simulink model "gauges"  (Simulink 7.5)
settings: Solver=ode45  StartTime=0.0  StopTime=10.0  RelTol=1e-3
undefined symbols (not defined in the file or in its folder): ECU565, motohawk_get_faults
libraries: MotoHawk_VDOGauge_lib x6, MotoHawk_lib x4, simulink x1
settings Model: Creator=Ethan  LastModifiedBy=Ethan

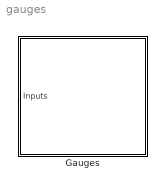
== system gauges ==
  Gauges : Subsystem

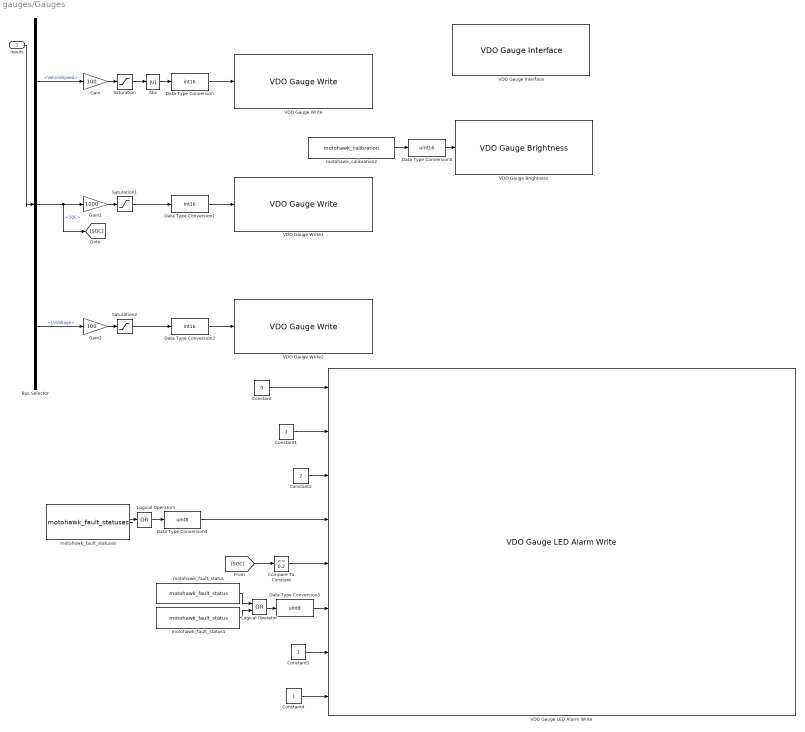
== system gauges/Gauges ==
  Inputs : Inport  OutDataType=sfix(16)  OutScaling=2^0
  Abs : Abs  OutDataType=fixdt(1, 16)  OutScaling=2^0
  Bus Selector : BusSelector  OutputSignals=VehicleSpeed,SOC,LVVoltage
  Compare To Constant : simulink/Logic and Bit Operations/Compare To Constant  SystemSampleTime=-1  relop=<=  const=0.2  LogicOutDataTypeMode=uint8
  Constant : Constant  Value=0  OutDataTypeMode=uint8  OutDataType=fixdt(1, 16)  OutScaling=2^0  OutDataTypeStr=uint8
  Constant1 : Constant  OutDataTypeMode=uint8  OutDataType=fixdt(1, 16)  OutScaling=2^0  OutDataTypeStr=uint8
  Constant2 : Constant  Value=2  OutDataTypeMode=uint8  OutDataType=fixdt(1, 16)  OutScaling=2^0  OutDataTypeStr=uint8
  Constant3 : Constant  OutDataTypeMode=uint8  OutDataType=fixdt(1, 16)  OutScaling=2^0  OutDataTypeStr=uint8
  Constant4 : Constant  OutDataTypeMode=uint8  OutDataType=fixdt(1, 16)  OutScaling=2^0  OutDataTypeStr=uint8
  Data Type Conversion : DataTypeConversion  OutDataTypeMode=int16  OutDataType=fixdt(1, 16)  OutScaling=2^0  OutDataTypeStr=int16
  Data Type Conversion1 : DataTypeConversion  OutDataTypeMode=int16  OutDataType=fixdt(1, 16)  OutScaling=2^0  OutDataTypeStr=int16
  Data Type Conversion2 : DataTypeConversion  OutDataTypeMode=int16  OutDataType=fixdt(1, 16)  OutScaling=2^0  OutDataTypeStr=int16
  Data Type Conversion3 : DataTypeConversion  OutDataTypeMode=uint8  OutDataType=fixdt(1, 16)  OutScaling=2^0  OutDataTypeStr=uint8
  Data Type Conversion4 : DataTypeConversion  OutDataTypeMode=uint8  OutDataType=fixdt(1, 16)  OutScaling=2^0  OutDataTypeStr=uint8
  Data Type Conversion5 : DataTypeConversion  OutDataTypeMode=uint16  OutDataType=fixdt(1, 16)  OutScaling=2^0  OutDataTypeStr=uint16
  Gain : Gain  Gain=100  ParameterDataType=fixdt(1, 16)  ParameterScaling=2^0  OutDataType=fixdt(1, 16)  OutScaling=2^0
  Gain1 : Gain  Gain=1000  ParameterDataType=fixdt(1, 16)  ParameterScaling=2^0  OutDataType=fixdt(1, 16)  OutScaling=2^0
  Gain2 : Gain  Gain=100  ParameterDataType=fixdt(1, 16)  ParameterScaling=2^0  OutDataType=fixdt(1, 16)  OutScaling=2^0
  Logical Operator : Logic  Operator=OR  AllPortsSameDT=off  OutDataTypeMode=boolean  LogicDataType=fixdt(0, 8)  OutDataTypeStr=boolean
  Logical Operator1 : Logic  Operator=OR  Inputs=1  AllPortsSameDT=off  OutDataTypeMode=boolean  LogicDataType=fixdt(0, 8)  OutDataTypeStr=boolean
  Saturation : Saturate  UpperLimit=100  LowerLimit=-100  OutDataType=fixdt(1, 16)  OutScaling=2^0
  Saturation1 : Saturate  UpperLimit=1000  LowerLimit=0  OutDataType=fixdt(1, 16)  OutScaling=2^0
  Saturation2 : Saturate  UpperLimit=20  LowerLimit=0  OutDataType=fixdt(1, 16)  OutScaling=2^0
  VDO Gauge Brightness : MotoHawk_VDOGauge_lib/VDO Gauge Brightness  nam='GaugeChain'  per=2000
  VDO Gauge Interface : MotoHawk_VDOGauge_lib/VDO Gauge Interface  nam='GaugeChain'  text_resource=(None)  code_resource=NONE  val_resource=-1  target=ECU565-128  dly=1600  queue_size=10  dyn_create=off
  VDO Gauge LED Alarm Write : MotoHawk_VDOGauge_lib/VDO Gauge LED Alarm Write  nam='GaugeChain'  pri=(None)
  VDO Gauge Write : MotoHawk_VDOGauge_lib/VDO Gauge Write  nam='GaugeChain'  res=Speed  pri=(None)
  VDO Gauge Write1 : MotoHawk_VDOGauge_lib/VDO Gauge Write  nam='GaugeChain'  res=Fuel Level  pri=(None)
  VDO Gauge Write2 : MotoHawk_VDOGauge_lib/VDO Gauge Write  nam='GaugeChain'  res=Voltage  pri=(None)
  motohawk_calibration2 : MotoHawk_lib/Calibration & Probing Blocks/motohawk_calibration  nam='VDO_Gauge_Brightness'  val=5  storage=Calibration  show_more=on  name_source=Use Parameter  data_type=uint16  read_level=1  write_level=1  ovr_cals=on  view_as=Number  enum_struct={'Disabled', 'Enabled'}  vector_style=Wide Row  use_help_units=off  help=''  units=''  use_header_enum=off  row_header_enum={}  col_header_enum={}  use_min_max=on  min_val=0  max_val=7  use_precision=off  precision=''  gain=1  offset=0  exp=1  use_mototune_group=on  mototune_group='Gauges'
  motohawk_fault_status : MotoHawk_lib/Fault Management Blocks/motohawk_fault_status  source=Lookup By Name  nam='LVVoltLow'  status=Active
  motohawk_fault_status1 : MotoHawk_lib/Fault Management Blocks/motohawk_fault_status  source=Lookup By Name  nam='LVVoltHigh'  status=Active
  motohawk_fault_statuses : MotoHawk_lib/Fault Management Blocks/motohawk_fault_statuses  nam=motohawk_get_faults(bdroot)  status=Active
  wires:
  Inputs/1 -> Bus Selector/1
  Bus Selector/1 -> Gain/1  "<VehicleSpeed>"
  Gain/1 -> Saturation/1
  Saturation/1 -> Abs/1
  Data Type Conversion/1 -> VDO Gauge Write/1
  Abs/1 -> Data Type Conversion/1
  Bus Selector/2 -> Gain1/1, [SOC]  "<SOC>"
  Gain1/1 -> Saturation1/1
  Saturation1/1 -> Data Type Conversion1/1
  Data Type Conversion1/1 -> VDO Gauge Write1/1
  Bus Selector/3 -> Gain2/1  "<LVVoltage>"
  Gain2/1 -> Saturation2/1
  Saturation2/1 -> Data Type Conversion2/1
  Data Type Conversion2/1 -> VDO Gauge Write2/1
  Constant/1 -> VDO Gauge LED Alarm Write/1
  Constant1/1 -> VDO Gauge LED Alarm Write/2
  Constant2/1 -> VDO Gauge LED Alarm Write/3
  motohawk_fault_status/1 -> Logical Operator/1
  motohawk_fault_status1/1 -> Logical Operator/2
  Logical Operator/1 -> Data Type Conversion3/1
  Data Type Conversion3/1 -> VDO Gauge LED Alarm Write/6
  motohawk_fault_statuses/1 -> Logical Operator1/1
  Logical Operator1/1 -> Data Type Conversion4/1
  Data Type Conversion4/1 -> VDO Gauge LED Alarm Write/4
  Compare To Constant/1 -> VDO Gauge LED Alarm Write/5
  [SOC] -> Compare To Constant/1
  Constant3/1 -> VDO Gauge LED Alarm Write/7
  Constant4/1 -> VDO Gauge LED Alarm Write/8
  motohawk_calibration2/1 -> Data Type Conversion5/1
  Data Type Conversion5/1 -> VDO Gauge Brightness/1
